simulink model "DIMR_ordinary"  (R2024b)
settings: Solver=daessc  StartTime=0.0  StopTime=60  RelTol=1e-3
values from neighbouring files (symbols this model uses):
  d_m0 = d_mn    (= 0)    [DIMR_main.m]
  d_m_cmd = 0.12787808985686    (= 0.127878089857)    [DIMR_main.m]
  dis_cmd = 0    [DIMR_main.m]
  jrk_cmd = 0.15    [DIMR_main.m]
  phi_cmd = 0*pi/180    (= 0)    [DIMR_main.m]
  ta = (vel_cmd-jrk_cmd*tt^2)/acc_cmd    (= 3.66666666667)    [DIMR_main.m]
  taz = z_vel_cmd/z_acc_cmd    (= 1.6)    [DIMR_main.m]
  tc = (x_cmd-2*(1/2*acc_cmd*ta^2+1/2*jrk_cmd*tt^2*ta+tt*vel_cmd))/vel_cmd    (= 10.6666666667)    [DIMR_main.m]
  tcz = (z_cmd-z_acc_cmd*taz^2)/z_vel_cmd    [DIMR_main.m]
  tcz2 = (z_cmd2-z_acc_cmd*taz^2)/z_vel_cmd    (= 0.9)    [DIMR_main.m]
  theta_f0 = -theta_p0    (= -0.024)    [DIMR_main.m]
  theta_f_cmd = 0.037940459    [DIMR_main.m]
  theta_p0 = theta_pn    (= 0.024)    [DIMR_main.m]
  theta_p_cmd = -0.037940459    [DIMR_main.m]
  ts = 15    [DIMR_main.m]
  ts2 = te+5    (= 39.3333333333)    [DIMR_main.m]
  tsz = 10    [DIMR_main.m]
  tsz2 = ts2    (= 39.3333333333)    [DIMR_main.m]
  tt = acc_cmd/jrk_cmd    (= 0.333333333333)    [DIMR_main.m]
  x_cmd = 3    [DIMR_main.m]
  z_0 = R_wo+L_bmy+L_my/2    [DIMR_main.m]
  z_acc_cmd = 0.05    [DIMR_main.m]
  z_cmd = 0.9-z_0    [DIMR_main.m]
  z_cmd2 = 0.9-0.7    (= 0.2)    [DIMR_main.m]
undefined symbols (not defined in the file or in its folder): Ac, Dc, DiscIntNeverNeededParam, dspblkCoreblockFVToolHelper, g, g_ext, g_fork, g_lift, g_reac, g_spado, g_yaw, gcbh, K_fd, K_fp, K_md, K_mp, K_pd, K_pp, K_wd, K_wi, K_wp, K_yd, K_yp, Kc, L_bg, L_bmx, L_bmy, L_bmz, L_bsx, L_bsy, L_bsz, L_by, L_ex, L_ey, L_ez, L_fg, L_fh, L_fx, L_fy, L_fz, L_lx, L_ly, L_lz, L_mg, L_mx, L_my, L_mz, L_wt, M_b, M_f, M_m, M_n11, M_n21, M_n22, M_n33, M_n44, Mc, N_f, N_w, omega_c ... (+10)
libraries: simulink x56, sm_lib x54, nesl_utility x12, slctrl_autotuning x1, slpidlib x1
(part 1 of 6)
settings Model: Creator=ITO  LastModifiedBy=Sergio Quintero
settings RTWCC: GPUComputeCapability=3.5

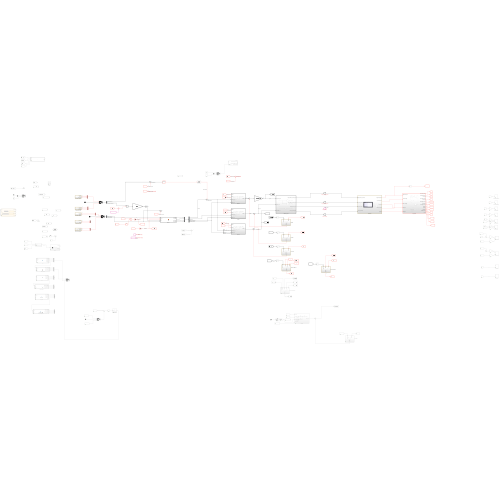
[thumbnail: Simulink's stored preview of the top-level diagram]
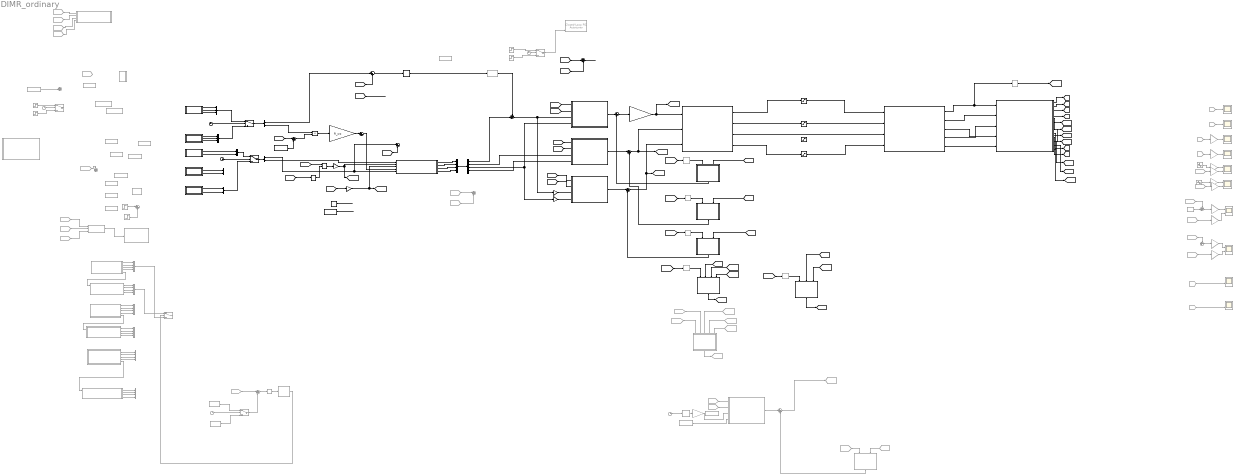
== system DIMR_ordinary ==
  Abs : Abs  Commented=on  SaturateOnIntegerOverflow=off
  Calc_states : Subsystem
  Chart : Stateflow chart  Commented=on  TreatAsAtomicUnit=on
  Clock{,1..2,5} (4 alike) : Clock  Commented=on
  Clock3 : Clock
  Clock6 : Clock
  Closed-Loop PID Autotuner : slctrl_autotuning/Closed-Loop PID Autotuner  Commented=on  PIDType=PID  PIDForm=Parallel  TimeDomain=discrete-time  DiscreteTs=T_control  TuningTs=0.2  UseTuningTs=off  IntegratorFormula=Forward Euler  FilterFormula=Forward Euler  ContinuousTs=0.02  Bandwidth=1  UseExternalWC=off  TargetPM=45  UseExternalPM=off  UseExternalAchievedPM=on  ExperimentMode=Superposition  PlantType=Stable  PlantSign=Positive  AmpSine=0.01  UseExternalAmpSine=off  UseExternalFRD=off  UseExternalU0=off  UseCompanion=off  NotDeployTuningModule=off  UsePLCCoder=off  OutputMode=control action + perturbation  BlockDataType=double  UseConnectedPID=on  blockpath=[]  tunedP=0  tunedI=0  tunedD=0  tunedN=100  tunedPM=0  EstimationWindowSize=3  UseExternalTuningParams=off  SingleMultiRateVariant=SingleSamplingRate  NumEstimationPeriods=4  NumSettlingPeriods=2  NumOfPRBSPeriod=1  PRBSSignalOrder=12  ExperimentModeVariant=VariantSuperimposed  OutputChoice=VariantCandD  ConvergenceCalcVariant=ConvSuperpositionPRBSVariant
      settings: LibrarySourceBlock=slctrlblks/Autotuning/Closed-Loop PID Autotuner
  Constant : Constant  Commented=on  Value=theta_p_cmd
  Constant1 : Constant  Commented=on  Value=phi_cmd
  Constant10 : Constant  Commented=on  Value=10.62*0.075
  Constant11 : Constant  Commented=on  Value=z_cmd
  Constant12 : Constant  Commented=on  Value=dis_cmd
  Constant13 : Constant  Commented=on  Value=0.0001
  Constant14 : Constant  Commented=on  Value=z_0
  Constant15 : Constant  Commented=on  Value=z_cmd
  Constant16 : Constant  Commented=on  Value=z_cmd2
  Constant17 : Constant  Value=M_b+M_f+M_m
  Constant18 : Constant  Commented=on  Value=theta_p0
  Constant19 : Constant  Value=5
  Constant2 : Constant  Commented=on  Value=theta_f_cmd
  Constant20 : Constant  Value=5*g*0.37
  Constant3 : Constant  Commented=on  Value=pi/2
  Constant4 : Constant  Commented=on  Value=pi/20
  Constant5 : Constant  Commented=on  Value=d_m_cmd
  Constant6 : Constant  Commented=on  Value=dis_cmd
  Constant7 : Constant  Commented=on  Value=0.298
  Constant8 : Constant  Commented=on  Value=0.6
  Constant9 : Constant  Commented=on  Value=0.019
  Cos : Trigonometry  Operator=cos
  Delay One Step{,1..5} (6 alike) : Delay  Commented=through  DelayLength=1
  Demux : Demux
  Demux1 : Demux  Outputs=3
  Demux2 : Demux  Outputs=2
  Divide : Product  Inputs=*/
  Fork DOB : Subsystem
  Fork PD : Subsystem
  Fork position : Scope  Commented=on  NumInputPorts=2
  Fork velocity : Scope  Commented=on  NumInputPorts=2
  From1 : From  Commented=on  GotoTag=dphi
  From10 : From  Commented=on  GotoTag=Yaw_input
  From{13,19,23,39} (4 alike) : From  Commented=on  GotoTag=dtheta_p
  From14 : From  Commented=on  GotoTag=d
  From15 : From  Commented=on  GotoTag=v
  From16 : From  Commented=on  GotoTag=phi
  From17 : From  Commented=on  GotoTag=dphi
  From{18,22,41,45,51,55} (6 alike) : From  Commented=on  GotoTag=theta_p
  From20 : From  Commented=on  GotoTag=theta_f
  From21 : From  Commented=on  GotoTag=dtheta_f
  From24 : From  Commented=on  GotoTag=X
  From25 : From  Commented=on  GotoTag=Y
  From30 : From  Commented=on  GotoTag=d
  From33 : From  Commented=on  GotoTag=t_ext_f
  From37 : From  Commented=on  GotoTag=Z_Fork
  From40 : From  Commented=on  GotoTag=Wheel_input
  From42 : From  Commented=on  GotoTag=theta_f
  From43 : From  Commented=on  GotoTag=d_m
  From44 : From  Commented=on  GotoTag=d_m
  From5 : From  Commented=on  GotoTag=phi
  From52 : From  Commented=on  GotoTag=d_m
  From53 : From  Commented=on  GotoTag=ml
  From54 : From  Commented=on  GotoTag=tl
  From58 : From  Commented=on  GotoTag=theta_f
  From6 : From  Commented=on  GotoTag=dphi
  Gain : Gain  Gain=-M_n11/(M_n21+M_n11)
  Gain{1..8,10..11} (10 alike) : Gain  Commented=on  Gain=180/pi
  Gain12 : Gain  Gain=1/g
  Gain13 : Gain  Gain=-1
  Gain14 : Gain  Gain=-1
  Gain15 : Gain  Gain=R_wo
  Gain16 : Gain  Gain=-1
  Gain9 : Gain  Commented=on  Gain=pi/20
  Goto11 : Goto  Commented=on  GotoTag=Yaw_input
  Goto19 : Goto  Commented=on  GotoTag=t_ext_p
  IK : MATLAB Function  Commented=on  TreatAsAtomicUnit=on
  IK1 : MATLAB Function  Commented=on  TreatAsAtomicUnit=on
  IK_simp : MATLAB Function  Commented=on  TreatAsAtomicUnit=on
  Lift DOB : Subsystem
  Lift PD : Subsystem
  MATLAB Function : MATLAB Function  Commented=on  TreatAsAtomicUnit=on
  Mux : Mux  Inputs=3
  Mux{1..4,8..9} (6 alike) : Mux  Commented=on
  Mux10 : Mux
  Mux11 : Mux  Inputs=2
  Mux5 : Mux  Inputs=2
  Mux6 : Mux  Inputs=3
  Mux7 : Mux  Inputs=2
  PID Controller1 : slpidlib/PID Controller  Controller=PID  Form=Parallel  TimeDomain=Discrete-time  UseExternalTs=off  SampleTime=T_control  IntegratorMethod=Forward Euler  FilterMethod=Forward Euler  ControllerParametersSource=internal  P=K_wp  I=K_wi  UseKiTs=off  D=K_wd  UseExternalDerivativeSource=off  N=100  UseFilter=off  TunerSelectOption=Transfer Function Based (PID Tuner App)  InitialConditionSource=internal  InitialConditionForIntegrator=0  InitialConditionForFilter=0  DifferentiatorICPrevScaledInput=0  ExternalReset=none  TrackingMode=off  Kt=1  LimitOutput=off  SatLimitsSource=internal  UpperSaturationLimit=inf  LowerSaturationLimit=-inf  LinearizeAsGain=on  AntiWindupMode=none  Kb=1  LimitIntegrator=off  UpperIntegratorSaturationLimit=inf  LowerIntegratorSaturationLimit=-inf  POutMin=[]  POutMax=[]  IOutMin=[]  IOutMax=[]  DOutMin=[]  DOutMax=[]  NOutMin=[]  NOutMax=[]  SumOutMin=[]  SumOutMax=[]  SaturationOutMin=[]  SaturationOutMax=[]  PParamMin=[]  PParamMax=[]  IParamMin=[]  IParamMax=[]  DParamMin=[]  DParamMax=[]  NParamMin=[]  NParamMax=[]  KbParamMin=[]  KbParamMax=[]  KtParamMin=[]  KtParamMax=[]  KbOutMin=[]  KbOutMax=[]  KtOutMin=[]  KtOutMax=[]  IntegratorOutMin=[]  IntegratorOutMax=[]  FilterOutMin=[]  FilterOutMax=[]  SumI1OutMin=[]  SumI1OutMax=[]  SumI2OutMin=[]  SumI2OutMax=[]  SumI3OutMin=[]  SumI3OutMax=[]  SumI4OutMin=[]  SumI4OutMax=[]  SumDOutMin=[]  SumDOutMax=[]  DifferentiatorOutMin=[]  DifferentiatorOutMax=[]  FilterDiffOutCoefMin=[]  FilterDiffOutCoefMax=[]  ReciprocalOutMin=[]  ReciprocalOutMax=[]  SumDenOutMin=[]  SumDenOutMax=[]  SumNumOutMin=[]  SumNumOutMax=[]  DivideOutMin=[]  DivideOutMax=[]  UdiffTsProdOutMin=[]  UdiffTsProdOutMax=[]  NTsProdOutMin=[]  NTsProdOutMax=[]  UintegralTsProdOutMin=[]  UintegralTsProdOutMax=[]  UngainTsProdOutMin=[]  UngainTsProdOutMax=[]  ClampingZeroOutDataTypeStr=Inherit: Inherit via back propagation  ClampingZeroOutMin=[]  ClampingZeroOutMax=[]  FilterDenConstantOutDataTypeStr=Inherit: Inherit via back propagation  FilterDenConstantOutMin=[]  FilterDenConstantOutMax=[]  PCopyOutDataTypeStr=Inherit: Inherit via back propagation  PCopyOutMin=[]  PCopyOutMax=[]  NCopyOutDataTypeStr=Inherit: Inherit via back propagation  NCopyOutMin=[]  NCopyOutMax=[]  IntegratorContinuousStateAttributes=''  IntegratorStateMustResolveToSignalObject=off  IntegratorRTWStateStorageClass=Auto  FilterContinuousStateAttributes=''  FilterStateMustResolveToSignalObject=off  FilterRTWStateStorageClass=Auto  ParallelPVariant=InternalParameters  IdealPVariant=Disabled  IVariant=InternalParameters  DVariant=InternalParameters  IntegratorVariant=Discrete  SatVariant=Disabled  AWVariant=Passthrough  PCopyVariant=Disabled  TRVariant=Disabled  FdbkBlocksVariant=Forward  IdealPFdbkVariant=Disabled  SatFdbkVariant=Disabled  DerivativeFilterVariant=Differentiator  NVariant=Passthrough  NCopyVariant=Disabled_SignalSpec  FilterICVariant=InternalICsDifferentiator  IntegratorICVariant=InternalICs  ExternalResetVariant=Disabled  TRSumVariant=Passthrough  SumFdbkVariant=Disabled  SumVariant=Sum_PID  TsampFilterVariant=InternalTs  TsampNgainVariant=Passthrough  TsampIntegralVariant=Disabled_SignalSpec  ExternalSaturationOutDataTypeStr=Inherit: Same as second input  DerivativeSourceVariant=ErrorSignal  PreIntVariant=InternalPreInt
  Pitch PD : Subsystem
  Pitch position : Scope  Commented=on  NumInputPorts=2
  Pitch velocity : Scope  Commented=on  NumInputPorts=2
  Plant model : Subsystem
  Product : Product
  RCC : Subsystem  Commented=on
  Rate Transition : RateTransition  Commented=on  OutPortSampleTime=T_control
  Reaction DOB fork : Subsystem
  Reaction DOB lift : Subsystem
  Reaction DOB pitch : Subsystem  Commented=on
  SPADO : Subsystem
  Sine Wave2 : Sin  Commented=on  Amplitude=10*pi/180  SampleTime=T_control
  Sine Wave3 : Sin  Commented=on  Amplitude=10*pi/180  Phase=pi/2  SampleTime=T_control
  Solution : MATLAB Function  TreatAsAtomicUnit=on
  State Control : Subsystem  Commented=on
  Step : Step  Commented=on  Time=12  SampleTime=0
  Step1 : Step  Commented=on  Time=20  After=-1  SampleTime=0
  Step2 : Step  Commented=on  Time=0  After=theta_p_cmd*3/2  SampleTime=0
  Step3 : Step  Commented=on  Time=0  After=theta_p_cmd/2  SampleTime=0
  Step4 : Step  Commented=on  Time=0  SampleTime=0
  Step5 : Step  Commented=on  Time=0  After=-1  SampleTime=0
  Subsystem : Subsystem  Commented=on
  Sum{,2,7,9,13,16} (6 alike) : Sum  Inputs=|++
  Sum1 : Sum  Commented=on  Inputs=|++
  Sum10 : Sum  Commented=on  Inputs=|++
  Sum11 : Sum  Commented=on  Inputs=|+-
  Sum12 : Sum  Inputs=|+-
  Sum15 : Sum  Inputs=|+-
  Sum17 : Sum  Commented=on  Inputs=|++
  Sum3 : Sum  Inputs=++|
  Sum4 : Sum  Commented=on  Inputs=-+|
  Sum5 : Sum  Commented=on  Inputs=-+|
  Sum6 : Sum  Commented=on  Inputs=-+|
  Sum8 : Sum  Commented=on  Inputs=++|
  Switch : Switch  Commented=on  Criteria=u2 > Threshold  Threshold=5  SaturateOnIntegerOverflow=off  InputSameDT=off
  Switch1 : Switch  Commented=on  Criteria=u2 > Threshold  Threshold=ts  SaturateOnIntegerOverflow=off  InputSameDT=off
  Switch2 : Switch  Commented=on  Criteria=u2 ~= 0  Threshold=z_cmd  SaturateOnIntegerOverflow=off  InputSameDT=off
  Switch3 : Switch  Commented=on  Criteria=u2 > Threshold  Threshold=30  SaturateOnIntegerOverflow=off  InputSameDT=off
  Switch4 : Switch  Criteria=u2 > Threshold  Threshold=ts2  SaturateOnIntegerOverflow=off  InputSameDT=off
  Switch5 : Switch  Criteria=u2 > Threshold  Threshold=tsz2  SaturateOnIntegerOverflow=off  InputSameDT=off
  Test : Subsystem  Commented=on
  Transfer Fcn Lead or Lag : simulink/Discrete/Transfer Fcn Lead or Lag  Commented=on  PoleZ=0.01  ZeroZ=0.5  ICPrevOutput=0.0  ICPrevInput=0.0  DoSatur=off
  Transfer Fcn Lead or Lag1 : simulink/Discrete/Transfer Fcn Lead or Lag  Commented=through  PoleZ=0.5  ZeroZ=0.55  ICPrevOutput=0.0  ICPrevInput=0.0  DoSatur=off
  Transform_input : Subsystem
  Translational position : Scope  Commented=on
  Translational velocity : Scope  Commented=on
  X movement profile : Subsystem
  X movement profile1 : Subsystem
  X position : Scope  Commented=on  NumInputPorts=2
  Y position : Scope  Commented=on  NumInputPorts=2
  Yaw DOB : Subsystem  Commented=on
  Yaw PD : Subsystem  Commented=on
  Yaw Position : Scope  Commented=on
  Yaw rate : Scope  Commented=on
  Z movement down-up : Subsystem
  Z movement profile : Subsystem
  Z movement profile1 : Subsystem
  simp_model : MATLAB Function  Commented=on  TreatAsAtomicUnit=on
  simp_model1 : MATLAB Function  Commented=on  TreatAsAtomicUnit=on
  simp_model_simp : MATLAB Function  Commented=on  TreatAsAtomicUnit=on
  torque_limit_fork : Saturate  UpperLimit=Torque_limit_f  LowerLimit=-Torque_limit_f
  torque_limit_left_wheel : Saturate  UpperLimit=Torque_limit_w  LowerLimit=-Torque_limit_w
  torque_limit_lift : Saturate  UpperLimit=Torque_limit_l  LowerLimit=-Torque_limit_l
  torque_limit_right_wheel : Saturate  UpperLimit=Torque_limit_w  LowerLimit=-Torque_limit_w
  wires:
  Plant model/4(Pitch_Euler_Angle) -> Calc_states/3(Pitch euler angle)
  Plant model/3(Fork_Angle) -> Calc_states/4(Fork angle)
  torque_limit_left_wheel/1 -> Plant model/2(Left_wheel_motor_torque)
  Transform_input/4(Fork_motor_torque_ref) -> torque_limit_fork/1
  torque_limit_right_wheel/1 -> Plant model/1(Right_wheel_motor_torque)
  torque_limit_fork/1 -> Plant model/4(Fork_motor_torque)
  Transform_input/1(Right_wheel_motor_torque_ref) -> torque_limit_right_wheel/1
  Transform_input/2(Left_wheel_motor_torque_ref) -> torque_limit_left_wheel/1
  Plant model/2(Left_Wheel_Angle) -> Calc_states/2(Left wheel angle)
  Gain/1 -> [Wheel_input], Transform_input/1(Wheel_torque_ref)  "Tp_ref"
  Pitch PD/1(Torque_ref) -> Sum/1  "Pitch PD"
  Sum/1 -> Gain/1
  Yaw PD/1(Torque_ref) -> Sum1/1
  Sum1/1 -> Goto11/1
  Yaw DOB/1(Est_dis) -> Sum1/2
  Fork PD/1(Torque_ref) -> Sum2/1
  Sum2/1 -> [Fork_input], Transform_input/3(Fork_torque_ref)  "Fork_torque"
  Calc_states/1(Translational position) -> [d]
  Calc_states/2(Translational velocity) -> [v]
  Calc_states/3(Yaw angle) -> [phi]
  Calc_states/4(Yaw angular velocity) -> [dphi]
  Calc_states/5(Pitch angle) -> [theta_p]
  Calc_states/6(Pitch angular velocity) -> [dtheta_p]
  Calc_states/7(Fork position) -> [theta_f]
  Calc_states/8(Fork angular velocity) -> [dtheta_f]
  Calc_states/9(X position) -> [X]
  Calc_states/10(Y position) -> [Y]
  From1/1 -> Yaw DOB/2(Velocity)
  [dtheta_p] -> Pitch PD/2(Velocity)  "Pitch ang vel"
  [theta_p] -> Pitch PD/1(Position)  "Pitch response"
  From5/1 -> Yaw PD/1(Position)
  From6/1 -> Yaw PD/2(Velocity)
  [theta_f] -> Fork PD/1(Position)  "Fork response"
  [dtheta_f] -> Fork PD/2(Velocity)
  From10/1 -> Yaw DOB/1(Input Torque)
  [theta_p] -> Cos/1
  From13/1 -> Sum4/1
  From14/1 -> Translational position/1  "res"
  From15/1 -> Translational velocity/1  "res"
  From16/1 -> Gain1/1
  From17/1 -> Gain2/1
  From18/1 -> Gain3/1
  From19/1 -> Gain4/1
  From20/1 -> Gain6/1
  From21/1 -> Gain8/1
  Sum5/1 -> Gain5/1
  Sum6/1 -> Gain7/1
  From22/1 -> Sum5/1
  Constant3/1 -> Sum5/2
  From23/1 -> Sum6/1
  Gain1/1 -> Yaw Position/1  "res"
  Gain2/1 -> Yaw rate/1  "res"
  Gain3/1 -> Pitch position/2  "res"
  Gain4/1 -> Pitch velocity/2  "res"
  Gain5/1 -> Fork position/1  "cmd"
  Gain6/1 -> Fork position/2  "res"
  Gain7/1 -> Fork velocity/1  "cmd"
  Gain8/1 -> Fork velocity/2  "res"
  Fork DOB/1(Est_dis) -> Sum2/2
  From24/1 -> X position/2  "res"
  From25/1 -> Y position/2  "res"
  Clock/1 -> Rate Transition/1
  Gain9/1 -> Yaw PD/3(Position_cmd)
  Rate Transition/1 -> Gain9/1
  Constant4/1 -> Yaw PD/4(Velocity_cmd)
  Gain10/1 -> Pitch position/1  "res"
  Sine Wave2/1 -> Gain10/1
  Gain11/1 -> Pitch velocity/1  "res"
  Sine Wave3/1 -> Gain11/1
  Lift PD/1(Torque_ref) -> Sum7/1
  Lift DOB/1(Est_dis) -> Sum7/2
  Sum7/1 -> [Lift_input], Transform_input/2(Lift_force_ref)  "Lift_force"
  Plant model/5(Lift_height) -> Calc_states/5(Lift height)
  Calc_states/11(Lift position) -> [d_m]
  Calc_states/12(Lift linear velocity) -> [dd_m]
  [d_m] -> Lift PD/1(Position)  "Lift response"
  [dd_m] -> Lift PD/2(Velocity)
  Transform_input/3(Lift_motor_torque_ref) -> Plant model/3(Lift_motor_torque)  "Control height"
  [dtheta_f] -> Reaction DOB fork/2(Velocity)
  [Fork_input] -> Delay One Step3/1  "Fork_in"
  Reaction DOB fork/1(Est_dis) -> [t_ext_f]  "t_ext_f"
  [theta_p] -> Reaction DOB fork/3(Theta_p)
  [theta_f] -> Reaction DOB fork/4(Theta_f)
  Step/1 -> Sum10/1
  Step1/1 -> Sum10/2
  Constant/1 -> Sum8/2
  Clock1/1 -> Switch/2
  Clock2/1 -> Switch1/2
  SPADO/1(Est_dis) -> Sum/2  "SPADO"
  Sum3/1 -> Gain13/1, Pitch PD/3(Position_cmd)  "Pitch reference"
  Step2/1 -> Switch/1
  Step3/1 -> Switch/3
  Gain14/1 -> Fork PD/4(Velocity_cmd)  "Fork velocity reference"
  Gain13/1 -> Fork PD/3(Position_cmd)  "Fork reference"
  Calc_states/13(Z Fork) -> [Z_Fork]
  [dtheta_p] -> SPADO/2(Velocity)
  [dtheta_f] -> Fork DOB/2(Velocity)
  [Wheel_input] -> Delay One Step/1
  [Fork_input] -> Delay One Step2/1
  [Lift_input] -> Delay One Step1/1
  [dd_m] -> Lift DOB/2(Velocity)
  From42/1 -> Reaction DOB pitch/4(Theta_f)
  From41/1 -> Reaction DOB pitch/3(Theta_p)
  Reaction DOB pitch/1(Est_dis) -> Goto19/1  "t_ext_p"
  From40/1 -> Reaction DOB pitch/1(Input Torque)
  From39/1 -> Reaction DOB pitch/2(Velocity)
  From43/1 -> Reaction DOB pitch/5(d_m)
  Gain15/1 -> Sum13/1
  [d] -> Sum12/2  "X Position response"
  Sum12/1 -> PID Controller1/1  "X Position error"
  From33/1 -> Subsystem/1(t)
  From44/1 -> Subsystem/2(d2)
  From45/1 -> Subsystem/3(th1)
  Subsystem/1(t_ext) -> RCC/1(t_ext)  "CoG_var"
  Gain16/1 -> [tl], Solution/3(tau)  "Estimated tl"
  IK/1(ik_theta1) -> Mux1/1
  IK/2(ik_delta2) -> Mux1/2
  IK/3(ik_dtheta1) -> Mux1/3
  IK/4(ik_ddelta2) -> Mux1/4
  simp_model/1(inv_cog_theta1) -> Mux4/1
  simp_model/2(inv_cog_delta2) -> Mux4/2
  simp_model/3(inv_cog_dtheta1) -> Mux4/3
  simp_model/4(inv_cog_ddelta2) -> Mux4/4
  [t_ext_f] -> Gain16/1
  [dd_m] -> Reaction DOB lift/2(Velocity)
  [Lift_input] -> Delay One Step4/1
  [theta_p] -> Reaction DOB lift/3(Pitch)
  Reaction DOB lift/1(Est_dis) -> [f_ext_m]
  [f_ext_m] -> Divide/1
  Cos/1 -> Divide/2
  Divide/1 -> Gain12/1
  Gain12/1 -> Solution/2(mass_l), [ml]  "Estimated ml"
  IK1/5(ik_lt) -> simp_model1/1(lt)
  IK1/1(ik_theta1) -> Mux2/1
  IK1/2(ik_delta2) -> Mux2/2
  IK1/3(ik_dtheta1) -> Mux2/3
  IK1/4(ik_ddelta2) -> Mux2/4
  simp_model1/1(inv_cog_theta1) -> Mux3/1
  simp_model1/2(inv_cog_delta2) -> Mux3/2
  simp_model1/3(inv_cog_dtheta1) -> Mux3/3
  simp_model1/4(inv_cog_ddelta2) -> Mux3/4
  IK/5(ik_lt) -> simp_model/1(lt)
  From37/1 -> Sum11/1  "Z Position response"
  Sum11/1 -> Abs/1
  Abs/1 -> State Control/1(Z Error)
  State Control/1(Out1) -> Switch2/2
  Constant15/1 -> Switch3/3
  Clock5/1 -> Switch3/2
  Constant16/1 -> Switch3/1
  Switch3/1 -> Sum11/2
  Clock3/1 -> Switch4/2
  X movement profile/1(Pos_cmd) -> Mux/1
  Mux/1 -> Switch4/3
  Switch4/1 -> Demux1/1
  Z movement profile/2(Vel_cmd) -> Mux5/2
  Z movement profile/1(Pos_cmd) -> Mux5/1
  Clock6/1 -> Switch5/2
  Switch5/1 -> Demux2/1
  X movement profile1/1(Pos_cmd) -> Mux6/1
  Mux6/1 -> Switch4/1
  Z movement profile1/1(Pos_cmd) -> Mux7/1
  Z movement profile1/2(Vel_cmd) -> Mux7/2
  Mux7/1 -> Switch5/1
  X movement profile1/3(Acc_cmd) -> Mux6/3
  X movement profile1/2(Vel_cmd) -> Mux6/2
  X movement profile/2(Vel_cmd) -> Mux/2
  X movement profile/3(Acc_cmd) -> Mux/3
  [v] -> ?  "X Velocity response"
  From51/1 -> MATLAB Function/1(thp)
  From52/1 -> MATLAB Function/2(dm)
  From53/1 -> MATLAB Function/3(ml)
  From54/1 -> MATLAB Function/4(tl)
  IK_simp/5(ik_lt) -> simp_model_simp/1(lt)
  IK_simp/1(ik_theta1) -> Mux8/1
  IK_simp/2(ik_delta2) -> Mux8/2
  IK_simp/3(ik_dtheta1) -> Mux8/3
  IK_simp/4(ik_ddelta2) -> Mux8/4
  simp_model_simp/1(inv_cog_theta1) -> Mux9/1
  simp_model_simp/2(inv_cog_delta2) -> Mux9/2
  simp_model_simp/3(inv_cog_dtheta1) -> Mux9/3
  simp_model_simp/4(inv_cog_ddelta2) -> Mux9/4
  Mux1/1 -> Switch2/3
  Mux4/1 -> Switch2/1
  [Z_Fork] -> Sum15/2  "Z Position response"
  Solution/2(sol_delta2) -> Mux10/2
  Solution/3(sol_dtheta1) -> Mux10/3
  Solution/4(sol_ddelta2) -> Mux10/4
  Mux10/1 -> Demux/1
  [ml] -> Sum16/1
  Constant17/1 -> Sum16/2
  Sum16/1 -> Product/2
  Product/1 -> Gain15/1
  Sum13/1 -> Solution/4(tau_w)  "tau_w"
  From55/1 -> Sum17/1  "Pitch response"
  From58/1 -> Sum17/2  "Fork response"
  Delay One Step/1 -> SPADO/1(Input Torque)
  Delay One Step1/1 -> Lift DOB/1(Input Torque)
  Delay One Step2/1 -> Fork DOB/1(Input Torque)
  Delay One Step3/1 -> Reaction DOB fork/1(Input Torque)
  Delay One Step4/1 -> Reaction DOB lift/1(Input Torque)
  Plant model/1(Right_Wheel_Angle) -> Delay One Step5/1, Calc_states/1(Right wheel angle)
  Delay One Step5/1 -> [theta_w]
  Demux/1 -> Sum3/2  "Pitch IK"
  Demux/2 -> Lift PD/3(Position_cmd)  "Lift reference"
  Demux/3 -> Pitch PD/4(Velocity_cmd), Gain14/1  "Pitch velocity reference"
  Demux/4 -> Lift PD/4(Velocity_cmd)  "Lift velocity reference"
  Demux2/1 -> Sum15/1, Solution/5(z)  "Z Position reference"
  Demux2/2 -> Solution/1(dz)  "Z Velocity reference"
  Demux1/3 -> Product/1  "X Acceleration reference"
  Demux1/1 -> Sum12/1  "X Position reference"
  Solution/1(sol_theta1) -> Mux10/1
  Transfer Fcn Lead or Lag1/1 -> Sum3/1  "Pitch controller"
  Switch1/1 -> Closed-Loop PID Autotuner/3
  Step5/1 -> Switch1/3
  Step4/1 -> Switch1/1
  PID Controller1/1 -> Transfer Fcn Lead or Lag1/1
  Z movement down-up/1(Pos_cmd) -> Mux11/1
  Z movement down-up/2(Vel_cmd) -> Mux11/2
  Mux11/1 -> Switch5/3
  [theta_p] -> Sum9/1  "Pitch response"
  [theta_f] -> Sum9/2  "Fork response"
  Sum9/1 -> ?  "Sum p+f"
  Constant19/1 -> ?  "Real ml"
  Constant20/1 -> ?  "Real tl"

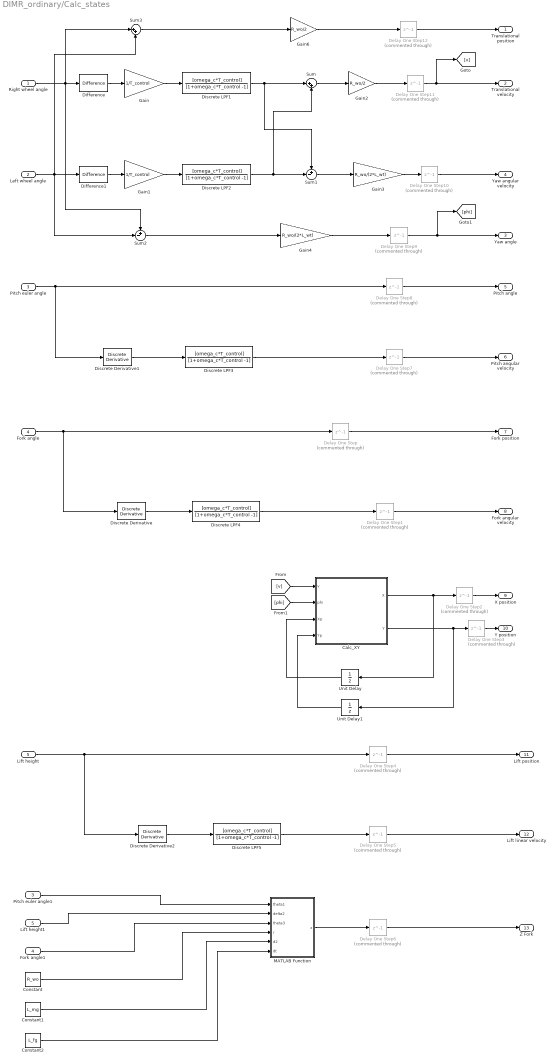
== system DIMR_ordinary/Calc_states ==
  Right wheel angle : Inport
  Left wheel angle : Inport  Port=2
  Pitch euler angle : Inport  Port=3
  Fork angle : Inport  Port=4
  Lift height : Inport  Port=5
  Calc_XY : MATLAB Function  TreatAsAtomicUnit=on
  Constant : Constant  Value=R_wo
  Constant1 : Constant  Value=L_mg
  Constant2 : Constant  Value=L_fg
  Delay One Step{,1..12} (13 alike) : Delay  Commented=through  DelayLength=1
  Difference : simulink/Discrete/Difference  ICPrevInput=0.0  OutMin=[]  OutMax=[]  OutDataType=fixdt(1, 16)  OutScaling=2^-10  DoSatur=off
  Difference1 : simulink/Discrete/Difference  ICPrevInput=0.0  OutMin=[]  OutMax=[]  OutDataType=fixdt(1, 16)  OutScaling=2^-10  DoSatur=off
  Discrete Derivative : simulink/Discrete/Discrete Derivative  gainval=1.0  ICPrevScaledInput=theta_f0/T_control  OutMin=[]  OutMax=[]  OutDataType=fixdt(1, 16)  OutScaling=2^-10  DoSatur=off
  Discrete Derivative1 : simulink/Discrete/Discrete Derivative  gainval=1.0  ICPrevScaledInput=theta_p0/T_control  OutMin=[]  OutMax=[]  OutDataType=fixdt(1, 16)  OutScaling=2^-10  DoSatur=off
  Discrete Derivative2 : simulink/Discrete/Discrete Derivative  gainval=1.0  ICPrevScaledInput=d_m0/T_control  OutMin=[]  OutMax=[]  OutDataType=fixdt(1, 16)  OutScaling=2^-10  DoSatur=off
  Discrete LPF1 : DiscreteFilter  LoadFcn=dspblkCoreblockFVToolHelper(gcbh,'load');  Numerator=[omega_c*T_control]  Denominator=[1+omega_c*T_control -1]
      settings: CopyFcn=dspblkCoreblockFVToolHelper(gcbh,'copy');  DeleteFcn=dspblkCoreblockFVToolHelper(gcbh,'close');  ModelCloseFcn=dspblkCoreblockFVToolHelper(gcbh,'close');  PreSaveFcn=dspblkCoreblockFVToolHelper(gcbh,'presave');  PostSaveFcn=dspblkCoreblockFVToolHelper(gcbh,'postsave');  CloseFcn=dspblkCoreblockFVToolHelper(gcbh,'close');
  Discrete LPF2 : DiscreteFilter  Numerator=[omega_c*T_control]  Denominator=[1+omega_c*T_control -1]
  Discrete LPF3 : DiscreteFilter  Numerator=[omega_c*T_control]  Denominator=[1+omega_c*T_control -1]
  Discrete LPF4 : DiscreteFilter  Numerator=[omega_c*T_control]  Denominator=[1+omega_c*T_control -1]
  Discrete LPF5 : DiscreteFilter  LoadFcn=dspblkCoreblockFVToolHelper(gcbh,'load');  Numerator=[omega_c*T_control]  Denominator=[1+omega_c*T_control -1]
      settings: CopyFcn=dspblkCoreblockFVToolHelper(gcbh,'copy');  DeleteFcn=dspblkCoreblockFVToolHelper(gcbh,'close');  ModelCloseFcn=dspblkCoreblockFVToolHelper(gcbh,'close');  PreSaveFcn=dspblkCoreblockFVToolHelper(gcbh,'presave');  PostSaveFcn=dspblkCoreblockFVToolHelper(gcbh,'postsave');  CloseFcn=dspblkCoreblockFVToolHelper(gcbh,'close');
  Fork angle1 : InportShadow  Port=4
  Gain : Gain  Gain=1/T_control
  Gain1 : Gain  Gain=1/T_control
  Gain2 : Gain  Gain=R_wo/2
  Gain3 : Gain  Gain=R_wo/(2*L_wt)
  Gain4 : Gain  Gain=R_wo/(2*L_wt)
  Gain6 : Gain  Gain=R_wo/2
  Lift height1 : InportShadow  Port=5
  MATLAB Function : MATLAB Function  TreatAsAtomicUnit=on
  Pitch euler angle1 : InportShadow  Port=3
  Sum : Sum  Inputs=|++
  Sum1 : Sum  Inputs=+-|
  Sum2 : Sum  Inputs=+-|
  Sum3 : Sum  Inputs=|++
  Unit Delay : UnitDelay  SampleTime=T_control  HasFrameUpgradeWarning=on
  Unit Delay1 : UnitDelay  SampleTime=T_control  HasFrameUpgradeWarning=on
  Translational position : Outport
  Translational velocity : Outport  Port=2
  Yaw angle : Outport  Port=3
  Yaw angular velocity : Outport  Port=4
  Pitch angle : Outport  Port=5
  Pitch angular velocity : Outport  Port=6
  Fork position : Outport  Port=7
  Fork angular velocity : Outport  Port=8
  X position : Outport  Port=9
  Y position : Outport  Port=10
  Lift position : Outport  Port=11
  Lift linear velocity : Outport  Port=12
  Z Fork : Outport  Port=13
  wires:
  Right wheel angle/1 -> Sum3/1, Sum2/1, Difference/1
  Difference/1 -> Gain/1
  Gain/1 -> Discrete LPF1/1
  Difference1/1 -> Gain1/1
  Gain1/1 -> Discrete LPF2/1
  Left wheel angle/1 -> Sum3/2, Sum2/2, Difference1/1
  Discrete LPF1/1 -> Sum/1, Sum1/1
  Discrete LPF2/1 -> Sum1/2, Sum/2
  Sum/1 -> Gain2/1
  Gain2/1 -> Delay One Step11/1
  Sum1/1 -> Gain3/1
  Gain3/1 -> Delay One Step10/1
  Sum2/1 -> Gain4/1
  Gain4/1 -> Delay One Step9/1
  Discrete Derivative1/1 -> Discrete LPF3/1
  Pitch euler angle/1 -> Delay One Step8/1, Discrete Derivative1/1
  Sum3/1 -> Gain6/1
  Gain6/1 -> Delay One Step12/1
  Discrete Derivative/1 -> Discrete LPF4/1
  Fork angle/1 -> Delay One Step/1, Discrete Derivative/1
  Discrete LPF4/1 -> Delay One Step1/1
  [v] -> Calc_XY/1(v)
  [phi] -> Calc_XY/2(phi)
  Calc_XY/1(X) -> Delay One Step2/1, Unit Delay/1
  Calc_XY/2(Y) -> Delay One Step3/1, Unit Delay1/1
  Unit Delay/1 -> Calc_XY/3(Xp)
  Unit Delay1/1 -> Calc_XY/4(Yp)
  Discrete LPF5/1 -> Delay One Step5/1
  Lift height/1 -> Delay One Step4/1, Discrete Derivative2/1
  Discrete Derivative2/1 -> Discrete LPF5/1
  Pitch euler angle1/1 -> MATLAB Function/1(theta1)
  Lift height1/1 -> MATLAB Function/2(delta2)
  Fork angle1/1 -> MATLAB Function/3(theta3)
  MATLAB Function/1(z) -> Delay One Step6/1
  Constant/1 -> MATLAB Function/4(r)
  Constant1/1 -> MATLAB Function/5(d2)
  Constant2/1 -> MATLAB Function/6(dt)
  Discrete LPF3/1 -> Delay One Step7/1
  Delay One Step7/1 -> Pitch angular velocity/1
  Delay One Step1/1 -> Fork angular velocity/1
  Delay One Step5/1 -> Lift linear velocity/1
  Delay One Step10/1 -> Yaw angular velocity/1
  Delay One Step11/1 -> Translational velocity/1, [v]
  Delay One Step12/1 -> Translational position/1
  Delay One Step9/1 -> [phi], Yaw angle/1
  Delay One Step8/1 -> Pitch angle/1
  Delay One Step/1 -> Fork position/1
  Delay One Step4/1 -> Lift position/1
  Delay One Step6/1 -> Z Fork/1
  Delay One Step2/1 -> X position/1
  Delay One Step3/1 -> Y position/1

== system DIMR_ordinary/Fork DOB ==
  Input Torque : Inport
  Velocity : Inport  Port=2
  Delay : Delay  Commented=through
  Discrete LPF1 : DiscreteFilter  LoadFcn=dspblkCoreblockFVToolHelper(gcbh,'load');  Numerator=[g_fork*T_control]  Denominator=[1+g_fork*T_control -1]
      settings: CopyFcn=dspblkCoreblockFVToolHelper(gcbh,'copy');  DeleteFcn=dspblkCoreblockFVToolHelper(gcbh,'close');  ModelCloseFcn=dspblkCoreblockFVToolHelper(gcbh,'close');  PreSaveFcn=dspblkCoreblockFVToolHelper(gcbh,'presave');  PostSaveFcn=dspblkCoreblockFVToolHelper(gcbh,'postsave');  CloseFcn=dspblkCoreblockFVToolHelper(gcbh,'close');
  Gain8 : Gain  Gain=g_fork*M_n44
  Sum5 : Sum  Inputs=+|+
  Sum6 : Sum  Inputs=|+-
  Est_dis : Outport
  wires:
  Velocity/1 -> Gain8/1
  Discrete LPF1/1 -> Sum6/1
  Gain8/1 -> Sum6/2, Sum5/2
  Input Torque/1 -> Sum5/1
  Sum6/1 -> Delay/1
  Sum5/1 -> Discrete LPF1/1
  Delay/1 -> Est_dis/1

== system DIMR_ordinary/Fork PD ==
  Position : Inport
  Velocity : Inport  Port=2
  Position_cmd : Inport  Port=3
  Velocity_cmd : Inport  Port=4
  Gain : Gain  Gain=K_fp
  Gain1 : Gain  Gain=K_fd
  Gain2 : Gain  Gain=M_n44
  Sum : Sum  Inputs=|+-
  Sum1 : Sum  Inputs=|+-
  Sum2 : Sum  Inputs=|++
  Torque_ref : Outport
  wires:
  Sum/1 -> Gain/1  "Fork error"
  Position/1 -> Sum/2
  Position_cmd/1 -> Sum/1
  Sum1/1 -> Gain1/1
  Velocity/1 -> Sum1/2
  Gain/1 -> Sum2/1
  Gain1/1 -> Sum2/2
  Sum2/1 -> Gain2/1
  Gain2/1 -> Torque_ref/1
  Velocity_cmd/1 -> Sum1/1

== system DIMR_ordinary/Lift DOB ==
  note: theta_p0
  Input Torque : Inport
  Velocity : Inport  Port=2
  Delay : Delay  Commented=through
  Discrete LPF1 : DiscreteFilter  LoadFcn=dspblkCoreblockFVToolHelper(gcbh,'load');  Numerator=[g_lift*T_control]  Denominator=[1+g_lift*T_control -1]
      settings: CopyFcn=dspblkCoreblockFVToolHelper(gcbh,'copy');  DeleteFcn=dspblkCoreblockFVToolHelper(gcbh,'close');  ModelCloseFcn=dspblkCoreblockFVToolHelper(gcbh,'close');  PreSaveFcn=dspblkCoreblockFVToolHelper(gcbh,'presave');  PostSaveFcn=dspblkCoreblockFVToolHelper(gcbh,'postsave');  CloseFcn=dspblkCoreblockFVToolHelper(gcbh,'close');
  Gain8 : Gain  Gain=g_lift*M_n33
  Sum5 : Sum  Inputs=+|+
  Sum6 : Sum  Inputs=|+-
  Est_dis : Outport
  wires:
  Sum5/1 -> Discrete LPF1/1
  Sum6/1 -> Delay/1
  Input Torque/1 -> Sum5/1
  Gain8/1 -> Sum5/2, Sum6/2
  Discrete LPF1/1 -> Sum6/1
  Velocity/1 -> Gain8/1
  Delay/1 -> Est_dis/1

== system DIMR_ordinary/Lift PD ==
  Position : Inport
  Velocity : Inport  Port=2
  Position_cmd : Inport  Port=3
  Velocity_cmd : Inport  Port=4
  Gain : Gain  Gain=K_mp
  Gain1 : Gain  Gain=K_md
  Gain2 : Gain  Gain=M_n33
  Sum : Sum  Inputs=|+-
  Sum1 : Sum  Inputs=|+-
  Sum2 : Sum  Inputs=|++
  Torque_ref : Outport
  wires:
  Velocity_cmd/1 -> Sum1/1
  Gain2/1 -> Torque_ref/1
  Sum2/1 -> Gain2/1
  Gain1/1 -> Sum2/2
  Gain/1 -> Sum2/1
  Velocity/1 -> Sum1/2
  Sum1/1 -> Gain1/1
  Position_cmd/1 -> Sum/1
  Position/1 -> Sum/2
  Sum/1 -> Gain/1  "Lift error"

== system DIMR_ordinary/Pitch PD ==
  Position : Inport
  Velocity : Inport  Port=2
  Position_cmd : Inport  Port=3
  Velocity_cmd : Inport  Port=4
  Gain : Gain  Gain=K_pp
  Gain1 : Gain  Gain=K_pd
  Gain2 : Gain  Gain=M_n22
  Sum : Sum  Inputs=|+-
  Sum1 : Sum  Inputs=|+-
  Sum2 : Sum  Inputs=|++
  Torque_ref : Outport
  wires:
  Sum/1 -> Gain/1  "Pitch Error"
  Position/1 -> Sum/2
  Position_cmd/1 -> Sum/1
  Sum1/1 -> Gain1/1
  Velocity_cmd/1 -> Sum1/1
  Velocity/1 -> Sum1/2
  Gain/1 -> Sum2/1
  Gain1/1 -> Sum2/2
  Sum2/1 -> Gain2/1
  Gain2/1 -> Torque_ref/1

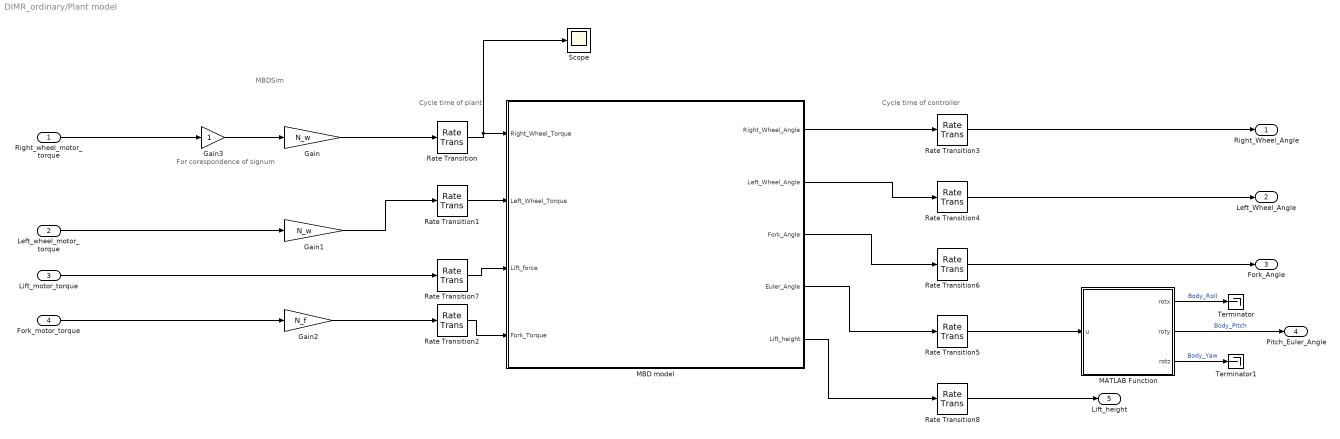
== system DIMR_ordinary/Plant model ==
  note: Cycle time of controller
  note: MBDSim
  note: For corespondence of signum
  note: Cycle time of plant
  Right_wheel_motor_torque : Inport
  Left_wheel_motor_torque : Inport  Port=2
  Lift_motor_torque : Inport  Port=3
  Fork_motor_torque : Inport  Port=4
  Gain : Gain  Gain=N_w
  Gain1 : Gain  Gain=N_w
  Gain2 : Gain  Gain=N_f
  Gain3 : Gain
  MATLAB Function : MATLAB Function  TreatAsAtomicUnit=on
  MBD model : Subsystem
  Rate Transition{,1..8} (9 alike) : RateTransition  OutPortSampleTime=T_control
  Scope : Scope
  Terminator : Terminator
  Terminator1 : Terminator
  Right_Wheel_Angle : Outport
  Left_Wheel_Angle : Outport  Port=2
  Fork_Angle : Outport  Port=3
  Pitch_Euler_Angle : Outport  Port=4
  Lift_height : Outport  Port=5
  wires:
  Rate Transition/1 -> Scope/1, MBD model/1(Right_Wheel_Torque)
  MBD model/3(Fork_Angle) -> Rate Transition6/1
  Gain3/1 -> Gain/1
  MBD model/1(Right_Wheel_Angle) -> Rate Transition3/1
  Rate Transition1/1 -> MBD model/2(Left_Wheel_Torque)
  Fork_motor_torque/1 -> Gain2/1
  MBD model/2(Left_Wheel_Angle) -> Rate Transition4/1
  Gain/1 -> Rate Transition/1
  MBD model/4(Euler_Angle) -> Rate Transition5/1
  Rate Transition2/1 -> MBD model/4(Fork_Torque)
  Gain2/1 -> Rate Transition2/1
  Gain1/1 -> Rate Transition1/1
  Left_wheel_motor_torque/1 -> Gain1/1
  Right_wheel_motor_torque/1 -> Gain3/1
  Rate Transition4/1 -> Left_Wheel_Angle/1
  Rate Transition3/1 -> Right_Wheel_Angle/1
  Rate Transition6/1 -> Fork_Angle/1
  MATLAB Function/1(rotx) -> Terminator/1  "Body_Roll"
  MATLAB Function/3(rotz) -> Terminator1/1  "Body_Yaw"
  Rate Transition5/1 -> MATLAB Function/1(u)
  MATLAB Function/2(roty) -> Pitch_Euler_Angle/1  "Body_Pitch"
  Lift_motor_torque/1 -> Rate Transition7/1
  Rate Transition8/1 -> Lift_height/1
  MBD model/5(Lift_height) -> Rate Transition8/1
  Rate Transition7/1 -> MBD model/3(Lift_force)

== system DIMR_ordinary/RCC ==
  t_ext : Inport
  Discrete Filter : DiscreteFilter  Commented=through  LoadFcn=dspblkCoreblockFVToolHelper(gcbh,'load');  Numerator=[1 -1]  Denominator=[1 g_ext*T_control-1]
      settings: CopyFcn=dspblkCoreblockFVToolHelper(gcbh,'copy');  DeleteFcn=dspblkCoreblockFVToolHelper(gcbh,'close');  ModelCloseFcn=dspblkCoreblockFVToolHelper(gcbh,'close');  PreSaveFcn=dspblkCoreblockFVToolHelper(gcbh,'presave');  PostSaveFcn=dspblkCoreblockFVToolHelper(gcbh,'postsave');  CloseFcn=dspblkCoreblockFVToolHelper(gcbh,'close');
  Discrete-Time Integrator : DiscreteIntegrator  SampleTime=T_control  ICPrevOutput=DiscIntNeverNeededParam  ICPrevScaledInput=DiscIntNeverNeededParam
  Discrete-Time Integrator1 : DiscreteIntegrator  SampleTime=T_control  ICPrevOutput=DiscIntNeverNeededParam  ICPrevScaledInput=DiscIntNeverNeededParam
  Gain12 : Gain  Gain=-Ac
  Gain13 : Gain  Gain=1/Mc
  Gain14 : Gain  Gain=Dc
  Gain15 : Gain  Gain=Kc
  Sum8 : Sum  Inputs=+-
  Sum9 : Sum  Inputs=|++
  theta_p : Outport
  dtheta_p : Outport  Port=2
  wires:
  Gain14/1 -> Sum9/2
  Discrete-Time Integrator1/1 -> theta_p/1, Gain15/1
  Gain13/1 -> Discrete-Time Integrator/1
  Sum8/1 -> Gain13/1
  Gain15/1 -> Sum9/1
  Sum9/1 -> Sum8/2
  Discrete-Time Integrator/1 -> Discrete-Time Integrator1/1, dtheta_p/1, Gain14/1
  Gain12/1 -> Sum8/1
  t_ext/1 -> Gain12/1

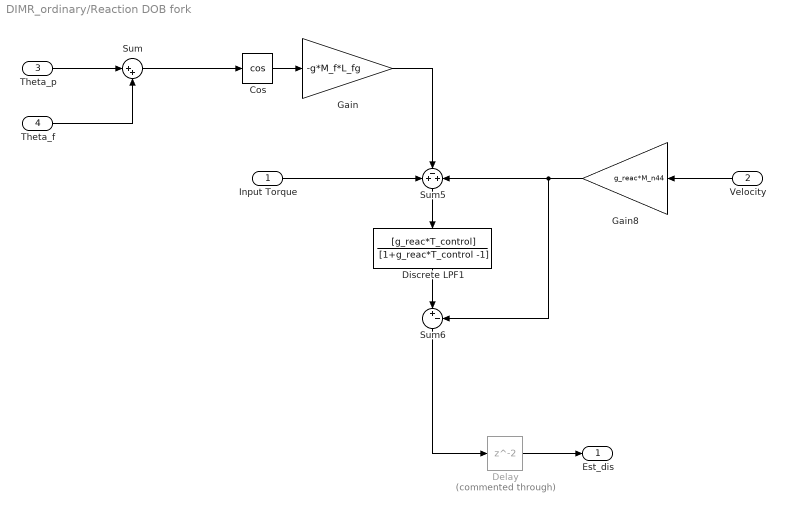
== system DIMR_ordinary/Reaction DOB fork ==
  Input Torque : Inport
  Velocity : Inport  Port=2
  Theta_p : Inport  Port=3
  Theta_f : Inport  Port=4
  Cos : Trigonometry  Operator=cos
  Delay : Delay  Commented=through
  Discrete LPF1 : DiscreteFilter  LoadFcn=dspblkCoreblockFVToolHelper(gcbh,'load');  Numerator=[g_reac*T_control]  Denominator=[1+g_reac*T_control -1]
      settings: CopyFcn=dspblkCoreblockFVToolHelper(gcbh,'copy');  DeleteFcn=dspblkCoreblockFVToolHelper(gcbh,'close');  ModelCloseFcn=dspblkCoreblockFVToolHelper(gcbh,'close');  PreSaveFcn=dspblkCoreblockFVToolHelper(gcbh,'presave');  PostSaveFcn=dspblkCoreblockFVToolHelper(gcbh,'postsave');  CloseFcn=dspblkCoreblockFVToolHelper(gcbh,'close');
  Gain : Gain  Gain=-g*M_f*L_fg
  Gain8 : Gain  Gain=g_reac*M_n44
  Sum : Sum  Inputs=|++
  Sum5 : Sum  Inputs=+-+
  Sum6 : Sum  Inputs=|+-
  Est_dis : Outport
  wires:
  Sum5/1 -> Discrete LPF1/1
  Sum6/1 -> Delay/1
  Input Torque/1 -> Sum5/1
  Gain8/1 -> Sum5/3, Sum6/2
  Discrete LPF1/1 -> Sum6/1
  Velocity/1 -> Gain8/1
  Cos/1 -> Gain/1
  Gain/1 -> Sum5/2
  Theta_p/1 -> Sum/1
  Theta_f/1 -> Sum/2
  Sum/1 -> Cos/1
  Delay/1 -> Est_dis/1

== system DIMR_ordinary/Reaction DOB lift ==
  Input Torque : Inport
  Velocity : Inport  Port=2
  Pitch : Inport  Port=3
  Cos : Trigonometry  Operator=cos
  Delay : Delay  Commented=through
  Discrete LPF1 : DiscreteFilter  LoadFcn=dspblkCoreblockFVToolHelper(gcbh,'load');  Numerator=[g_reac*T_control]  Denominator=[1+g_reac*T_control -1]
      settings: CopyFcn=dspblkCoreblockFVToolHelper(gcbh,'copy');  DeleteFcn=dspblkCoreblockFVToolHelper(gcbh,'close');  ModelCloseFcn=dspblkCoreblockFVToolHelper(gcbh,'close');  PreSaveFcn=dspblkCoreblockFVToolHelper(gcbh,'presave');  PostSaveFcn=dspblkCoreblockFVToolHelper(gcbh,'postsave');  CloseFcn=dspblkCoreblockFVToolHelper(gcbh,'close');
  Gain : Gain  Gain=g*(M_f+M_m)
  Gain8 : Gain  Gain=g_reac*M_n33
  Sum5 : Sum  Inputs=+-+
  Sum6 : Sum  Inputs=|+-
  Est_dis : Outport
  wires:
  Velocity/1 -> Gain8/1
  Discrete LPF1/1 -> Sum6/1
  Gain8/1 -> Sum5/3, Sum6/2
  Input Torque/1 -> Sum5/1
  Sum6/1 -> Delay/1
  Sum5/1 -> Discrete LPF1/1
  Pitch/1 -> Cos/1
  Cos/1 -> Gain/1
  Gain/1 -> Sum5/2
  Delay/1 -> Est_dis/1

== system DIMR_ordinary/Reaction DOB pitch ==
  Input Torque : Inport
  Velocity : Inport  Port=2
  Theta_p : Inport  Port=3
  Theta_f : Inport  Port=4
  d_m : Inport  Port=5
  Discrete LPF1 : DiscreteFilter  LoadFcn=dspblkCoreblockFVToolHelper(gcbh,'load');  Numerator=[g_reac*T_control]  Denominator=[1+g_reac*T_control -1]
      settings: CopyFcn=dspblkCoreblockFVToolHelper(gcbh,'copy');  DeleteFcn=dspblkCoreblockFVToolHelper(gcbh,'close');  ModelCloseFcn=dspblkCoreblockFVToolHelper(gcbh,'close');  PreSaveFcn=dspblkCoreblockFVToolHelper(gcbh,'presave');  PostSaveFcn=dspblkCoreblockFVToolHelper(gcbh,'postsave');  CloseFcn=dspblkCoreblockFVToolHelper(gcbh,'close');
  Gain8 : Gain  Gain=g_reac*M_n22
  Gravity : Subsystem
  Sum5 : Sum  Inputs=--+
  Sum6 : Sum  Inputs=|+-
  Est_dis : Outport
  wires:
  Velocity/1 -> Gain8/1
  Discrete LPF1/1 -> Sum6/1
  Gain8/1 -> Sum6/2, Sum5/3
  Input Torque/1 -> Sum5/1
  Sum6/1 -> Est_dis/1
  Sum5/1 -> Discrete LPF1/1
  Theta_p/1 -> Gravity/1(Theta_p)
  d_m/1 -> Gravity/2(d_m)
  Theta_f/1 -> Gravity/3(Theta_f)
  Gravity/1(g2) -> Sum5/2

== system DIMR_ordinary/SPADO ==
  Input Torque : Inport
  Velocity : Inport  Port=2
  Delay : Delay  Commented=through
  Discrete LPF1 : DiscreteFilter  Numerator=[g_spado*T_control]  Denominator=[1+g_spado*T_control -1]
  Gain1 : Gain  Gain=(M_n21+M_n11)/M_n11
  Gain8 : Gain  Gain=g_spado*M_n22
  Sum5 : Sum  Inputs=-|+
  Sum6 : Sum  Inputs=|+-
  Est_dis : Outport
  wires:
  Velocity/1 -> Gain8/1
  Discrete LPF1/1 -> Sum6/1
  Gain8/1 -> Sum6/2, Sum5/2
  Sum5/1 -> Discrete LPF1/1
  Gain1/1 -> Sum5/1
  Input Torque/1 -> Gain1/1
  Delay/1 -> Est_dis/1
  Sum6/1 -> Delay/1

== system DIMR_ordinary/State Control ==
  Z Error : Inport
  Compare To Constant : simulink/Logic and Bit Operations/Compare To Constant  relop=<=  const=0.01  OutDataTypeStr=boolean
  Out1 : Outport
  wires:
  Compare To Constant/1 -> Out1/1
  Z Error/1 -> Compare To Constant/1

== system DIMR_ordinary/Subsystem ==
  t : Inport
  d2 : Inport  Port=2
  th1 : Inport  Port=3
  Add : Sum  Inputs=+++
  Gain : Gain  Gain=1/L_fg
  Gain1 : Gain  Gain=L_mg
  Gain2 : Gain  Gain=-1/g
  Product : Product  Inputs=3
  Product1 : Product
  Sin : Trigonometry
  t_ext : Outport
  wires:
  th1/1 -> Sin/1
  Sin/1 -> Gain1/1, Product/2
  Product/1 -> Add/2
  d2/1 -> Product/1
  Gain/1 -> Product1/1, Product/3  "m"
  Gain1/1 -> Product1/2
  Product1/1 -> Add/3
  Add/1 -> t_ext/1
  t/1 -> Gain2/1
  Gain2/1 -> Gain/1, Add/1

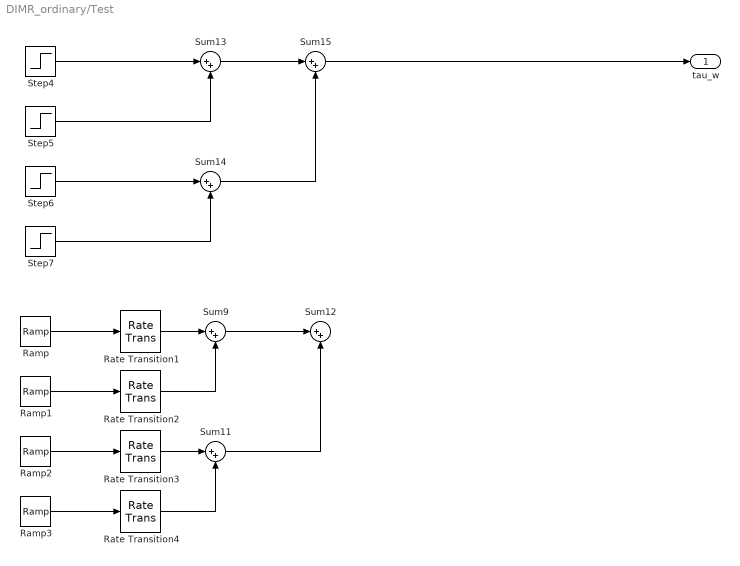
== system DIMR_ordinary/Test ==
  Ramp : simulink/Sources/Ramp  slope=9.6/0.1  start=7  InitialOutput=0.001
  Ramp1 : simulink/Sources/Ramp  slope=-9.6/0.1  start=7.1  InitialOutput=0.001
  Ramp2 : simulink/Sources/Ramp  slope=-9.6/0.1  start=9  InitialOutput=0.001
  Ramp3 : simulink/Sources/Ramp  slope=9.6/0.1  start=9.1  InitialOutput=0.001
  Rate Transition{1..4} (4 alike) : RateTransition  OutPortSampleTime=T_control
  Step4 : Step  Time=7  Before=0.001  After=0.8  SampleTime=T_control
  Step5 : Step  Time=9  After=-0.8+0.001  SampleTime=T_control
  Step6 : Step  Time=14  After=-0.8-0.001  SampleTime=T_control
  Step7 : Step  Time=16  After=0.8+0.001  SampleTime=T_control
  Sum{9,11..15} (6 alike) : Sum  Inputs=|++
  tau_w : Outport
  wires:
  Step4/1 -> Sum13/1
  Step5/1 -> Sum13/2
  Step7/1 -> Sum14/2
  Step6/1 -> Sum14/1
  Sum13/1 -> Sum15/1
  Sum14/1 -> Sum15/2
  Rate Transition1/1 -> Sum9/1
  Ramp2/1 -> Rate Transition3/1
  Ramp/1 -> Rate Transition1/1
  Sum11/1 -> Sum12/2
  Ramp1/1 -> Rate Transition2/1
  Rate Transition2/1 -> Sum9/2
  Ramp3/1 -> Rate Transition4/1
  Rate Transition4/1 -> Sum11/2
  Sum9/1 -> Sum12/1
  Rate Transition3/1 -> Sum11/1
  Sum15/1 -> tau_w/1

== system DIMR_ordinary/Transform_input ==
  Wheel_torque_ref : Inport
  Lift_force_ref : Inport  Port=2
  Fork_torque_ref : Inport  Port=3
  Gain : Gain  Gain=1/N_f
  Gain1 : Gain  Gain=R_wo/(2*N_w)
  Gain3 : Gain  Gain=R_wo/(2*N_w)
  Right_wheel_motor_torque_ref : Outport
  Left_wheel_motor_torque_ref : Outport  Port=2
  Lift_motor_torque_ref : Outport  Port=3
  Fork_motor_torque_ref : Outport  Port=4
  wires:
  Fork_torque_ref/1 -> Gain/1
  Gain/1 -> Fork_motor_torque_ref/1
  Gain1/1 -> Right_wheel_motor_torque_ref/1
  Wheel_torque_ref/1 -> Gain3/1, Gain1/1
  Gain3/1 -> Left_wheel_motor_torque_ref/1
  Lift_force_ref/1 -> Lift_motor_torque_ref/1

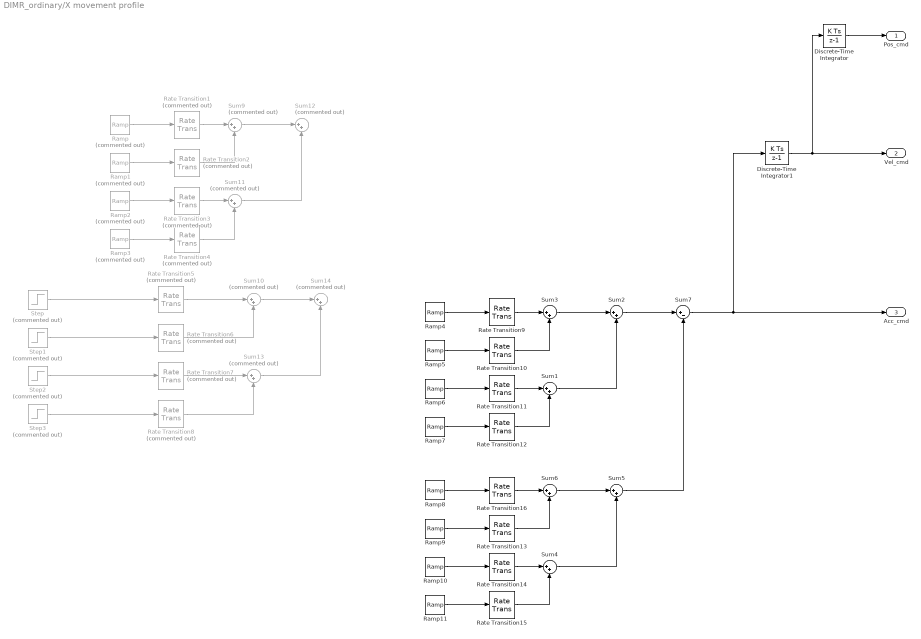
== system DIMR_ordinary/X movement profile ==
  Discrete-Time Integrator : DiscreteIntegrator  SampleTime=T_control  ICPrevOutput=DiscIntNeverNeededParam  ICPrevScaledInput=DiscIntNeverNeededParam
  Discrete-Time Integrator1 : DiscreteIntegrator  SampleTime=T_control  ICPrevOutput=DiscIntNeverNeededParam  ICPrevScaledInput=DiscIntNeverNeededParam
  Ramp : simulink/Sources/Ramp  Commented=on  slope=0.3/2  start=7  InitialOutput=0
  Ramp1 : simulink/Sources/Ramp  Commented=on  slope=-0.3/2  start=9  InitialOutput=0
  Ramp10 : simulink/Sources/Ramp  slope=-jrk_cmd  start=ts+2*ta+3*tt+tc  InitialOutput=0
  Ramp11 : simulink/Sources/Ramp  slope=jrk_cmd  start=ts+2*ta+4*tt+tc  InitialOutput=0
  Ramp2 : simulink/Sources/Ramp  Commented=on  slope=-0.3/2  start=14  InitialOutput=0
  Ramp3 : simulink/Sources/Ramp  Commented=on  slope=0.3/2  start=16  InitialOutput=0
  Ramp4 : simulink/Sources/Ramp  slope=jrk_cmd  start=ts  InitialOutput=0
  Ramp5 : simulink/Sources/Ramp  slope=-jrk_cmd  start=ts+tt  InitialOutput=0
  Ramp6 : simulink/Sources/Ramp  slope=-jrk_cmd  start=ts+tt+ta  InitialOutput=0
  Ramp7 : simulink/Sources/Ramp  slope=jrk_cmd  start=ts+ta+2*tt  InitialOutput=0
  Ramp8 : simulink/Sources/Ramp  slope=jrk_cmd  start=ts+ta+2*tt+tc  InitialOutput=0
  Ramp9 : simulink/Sources/Ramp  slope=-jrk_cmd  start=ts+ta+3*tt+tc  InitialOutput=0
  Rate Transition{1..8} (8 alike) : RateTransition  Commented=on  OutPortSampleTime=T_control
  Rate Transition{9..16} (8 alike) : RateTransition  OutPortSampleTime=T_control
  Step : Step  Commented=on  Time=7  After=0.3/2  SampleTime=T_control
  Step1 : Step  Commented=on  Time=9  After=-0.3/2  SampleTime=T_control
  Step2 : Step  Commented=on  Time=14  After=-0.3/2  SampleTime=T_control
  Step3 : Step  Commented=on  Time=16  After=0.3/2  SampleTime=T_control
  Sum{1..6} (6 alike) : Sum  Inputs=|++
  Sum{9..14} (6 alike) : Sum  Commented=on  Inputs=|++
  Sum7 : Sum  Inputs=|+-
  Pos_cmd : Outport
  Vel_cmd : Outport  Port=2
  Acc_cmd : Outport  Port=3
  wires:
  Ramp3/1 -> Rate Transition4/1
  Ramp2/1 -> Rate Transition3/1
  Sum10/1 -> Sum14/1
  Rate Transition2/1 -> Sum9/2
  Rate Transition3/1 -> Sum11/1
  Rate Transition1/1 -> Sum9/1
  Ramp/1 -> Rate Transition1/1
  Sum13/1 -> Sum14/2
  Sum11/1 -> Sum12/2
  Ramp1/1 -> Rate Transition2/1
  Sum9/1 -> Sum12/1
  Rate Transition4/1 -> Sum11/2
  Discrete-Time Integrator/1 -> Pos_cmd/1
  Step2/1 -> Rate Transition7/1
  Step/1 -> Rate Transition5/1
  Step1/1 -> Rate Transition6/1
  Step3/1 -> Rate Transition8/1
  Rate Transition7/1 -> Sum13/1
  Rate Transition8/1 -> Sum13/2
  Rate Transition6/1 -> Sum10/2
  Rate Transition5/1 -> Sum10/1
  Ramp6/1 -> Rate Transition11/1
  Sum3/1 -> Sum2/1
  Rate Transition12/1 -> Sum1/2
  Ramp4/1 -> Rate Transition9/1
  Sum1/1 -> Sum2/2
  Ramp7/1 -> Rate Transition12/1
  Rate Transition9/1 -> Sum3/1
  Rate Transition11/1 -> Sum1/1
  Ramp5/1 -> Rate Transition10/1
  Rate Transition10/1 -> Sum3/2
  Discrete-Time Integrator1/1 -> Discrete-Time Integrator/1, Vel_cmd/1
  Rate Transition13/1 -> Sum6/2
  Ramp9/1 -> Rate Transition13/1
  Rate Transition15/1 -> Sum4/2
  Ramp8/1 -> Rate Transition16/1
  Ramp11/1 -> Rate Transition15/1
  Rate Transition14/1 -> Sum4/1
  Sum4/1 -> Sum5/2
  Ramp10/1 -> Rate Transition14/1
  Sum6/1 -> Sum5/1
  Rate Transition16/1 -> Sum6/1
  Sum2/1 -> Sum7/1
  Sum7/1 -> Discrete-Time Integrator1/1, Acc_cmd/1
  Sum5/1 -> Sum7/2

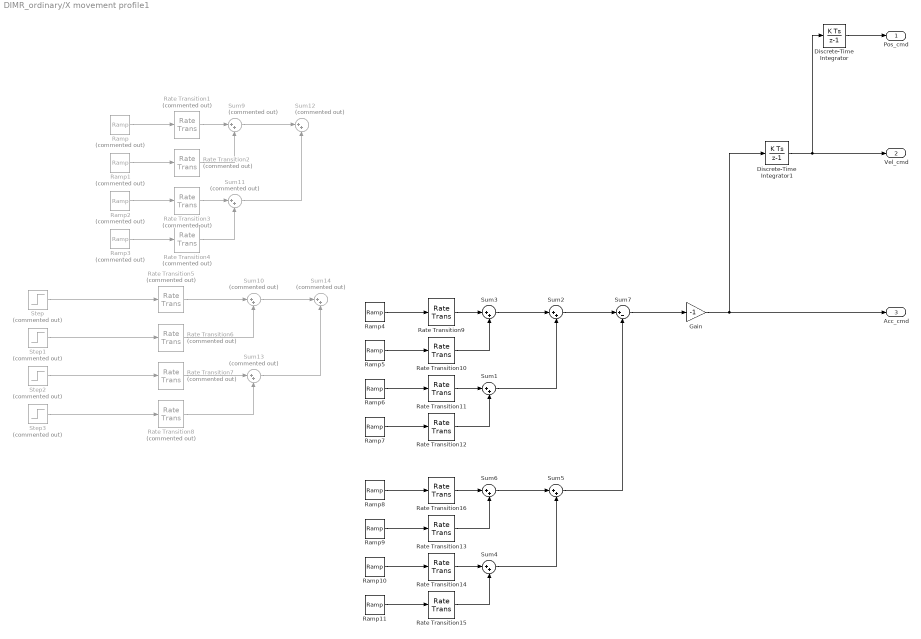
== system DIMR_ordinary/X movement profile1 ==
  Discrete-Time Integrator : DiscreteIntegrator  InitialCondition=x_cmd  SampleTime=T_control  ICPrevOutput=DiscIntNeverNeededParam  ICPrevScaledInput=DiscIntNeverNeededParam
  Discrete-Time Integrator1 : DiscreteIntegrator  SampleTime=T_control  ICPrevOutput=DiscIntNeverNeededParam  ICPrevScaledInput=DiscIntNeverNeededParam
  Gain : Gain  Gain=-1
  Ramp : simulink/Sources/Ramp  Commented=on  slope=0.3/2  start=7  InitialOutput=0
  Ramp1 : simulink/Sources/Ramp  Commented=on  slope=-0.3/2  start=9  InitialOutput=0
  Ramp10 : simulink/Sources/Ramp  slope=-jrk_cmd  start=ts2+2*ta+3*tt+tc  InitialOutput=0
  Ramp11 : simulink/Sources/Ramp  slope=jrk_cmd  start=ts2+2*ta+4*tt+tc  InitialOutput=0
  Ramp2 : simulink/Sources/Ramp  Commented=on  slope=-0.3/2  start=14  InitialOutput=0
  Ramp3 : simulink/Sources/Ramp  Commented=on  slope=0.3/2  start=16  InitialOutput=0
  Ramp4 : simulink/Sources/Ramp  slope=jrk_cmd  start=ts2  InitialOutput=0
  Ramp5 : simulink/Sources/Ramp  slope=-jrk_cmd  start=ts2+tt  InitialOutput=0
  Ramp6 : simulink/Sources/Ramp  slope=-jrk_cmd  start=ts2+tt+ta  InitialOutput=0
  Ramp7 : simulink/Sources/Ramp  slope=jrk_cmd  start=ts2+ta+2*tt  InitialOutput=0
  Ramp8 : simulink/Sources/Ramp  slope=jrk_cmd  start=ts2+ta+2*tt+tc  InitialOutput=0
  Ramp9 : simulink/Sources/Ramp  slope=-jrk_cmd  start=ts2+ta+3*tt+tc  InitialOutput=0
  Rate Transition{1..8} (8 alike) : RateTransition  Commented=on  OutPortSampleTime=T_control
  Rate Transition{9..16} (8 alike) : RateTransition  OutPortSampleTime=T_control
  Step : Step  Commented=on  Time=7  After=0.3/2  SampleTime=T_control
  Step1 : Step  Commented=on  Time=9  After=-0.3/2  SampleTime=T_control
  Step2 : Step  Commented=on  Time=14  After=-0.3/2  SampleTime=T_control
  Step3 : Step  Commented=on  Time=16  After=0.3/2  SampleTime=T_control
  Sum{1..6} (6 alike) : Sum  Inputs=|++
  Sum{9..14} (6 alike) : Sum  Commented=on  Inputs=|++
  Sum7 : Sum  Inputs=|+-
  Pos_cmd : Outport
  Vel_cmd : Outport  Port=2
  Acc_cmd : Outport  Port=3
  wires:
  Discrete-Time Integrator1/1 -> Vel_cmd/1, Discrete-Time Integrator/1
  Rate Transition5/1 -> Sum10/1
  Rate Transition6/1 -> Sum10/2
  Rate Transition8/1 -> Sum13/2
  Rate Transition7/1 -> Sum13/1
  Step3/1 -> Rate Transition8/1
  Step1/1 -> Rate Transition6/1
  Step/1 -> Rate Transition5/1
  Step2/1 -> Rate Transition7/1
  Discrete-Time Integrator/1 -> Pos_cmd/1
  Rate Transition4/1 -> Sum11/2
  Sum9/1 -> Sum12/1
  Ramp1/1 -> Rate Transition2/1
  Sum11/1 -> Sum12/2
  Sum13/1 -> Sum14/2
  Ramp/1 -> Rate Transition1/1
  Rate Transition1/1 -> Sum9/1
  Rate Transition3/1 -> Sum11/1
  Rate Transition2/1 -> Sum9/2
  Sum10/1 -> Sum14/1
  Ramp2/1 -> Rate Transition3/1
  Ramp3/1 -> Rate Transition4/1
  Gain/1 -> Discrete-Time Integrator1/1, Acc_cmd/1
  Rate Transition14/1 -> Sum4/1
  Sum1/1 -> Sum2/2
  Sum5/1 -> Sum7/2
  Ramp11/1 -> Rate Transition15/1
  Ramp8/1 -> Rate Transition16/1
  Rate Transition10/1 -> Sum3/2
  Sum6/1 -> Sum5/1
  Sum3/1 -> Sum2/1
  Ramp7/1 -> Rate Transition12/1
  Sum2/1 -> Sum7/1
  Rate Transition11/1 -> Sum1/1
  Ramp10/1 -> Rate Transition14/1
  Rate Transition12/1 -> Sum1/2
  Rate Transition9/1 -> Sum3/1
  Ramp9/1 -> Rate Transition13/1
  Ramp4/1 -> Rate Transition9/1
  Sum4/1 -> Sum5/2
  Rate Transition16/1 -> Sum6/1
  Ramp5/1 -> Rate Transition10/1
  Rate Transition13/1 -> Sum6/2
  Ramp6/1 -> Rate Transition11/1
  Rate Transition15/1 -> Sum4/2
  Sum7/1 -> Gain/1

== system DIMR_ordinary/Yaw DOB ==
  Input Torque : Inport
  Velocity : Inport  Port=2
  Discrete LPF1 : DiscreteFilter  Numerator=[g_yaw*T_control]  Denominator=[1+g_yaw*T_control -1]
  Gain8 : Gain  Gain=g_yaw*M_n22
  Scope5 : Scope
  Sum5 : Sum  Inputs=+|+
  Sum6 : Sum  Inputs=|+-
  Est_dis : Outport
  wires:
  Velocity/1 -> Gain8/1
  Discrete LPF1/1 -> Sum6/1
  Gain8/1 -> Sum6/2, Sum5/2
  Input Torque/1 -> Sum5/1
  Sum6/1 -> Est_dis/1, Scope5/1
  Sum5/1 -> Discrete LPF1/1

== system DIMR_ordinary/Yaw PD ==
  Position : Inport
  Velocity : Inport  Port=2
  Position_cmd : Inport  Port=3
  Velocity_cmd : Inport  Port=4
  Gain : Gain  Gain=K_yp
  Gain1 : Gain  Gain=K_yd
  Gain2 : Gain  Gain=M_n22
  Sum : Sum  Inputs=|+-
  Sum1 : Sum  Inputs=|+-
  Sum2 : Sum  Inputs=|++
  Torque_ref : Outport
  wires:
  Sum/1 -> Gain/1
  Position/1 -> Sum/2
  Position_cmd/1 -> Sum/1
  Sum1/1 -> Gain1/1
  Velocity_cmd/1 -> Sum1/1
  Velocity/1 -> Sum1/2
  Gain/1 -> Sum2/1
  Gain1/1 -> Sum2/2
  Sum2/1 -> Gain2/1
  Gain2/1 -> Torque_ref/1
